simulink model "elaborated_design"  (Simulink 7.0)
settings: Solver=ode45  SolverMode=SingleTasking  StartTime=0.0  StopTime=24/3000  RelTol=1e-6
PreLoadFcn:
  | load one_stage.mat
  | load multi_stage.mat
  | generate_fir_lut
undefined symbols (not defined in the file or in its folder): hm, lut_matrix
libraries: simulink x9, dspmlti4 x4, simulink_extras x2, dspsigops x1
(part 2 of 2)

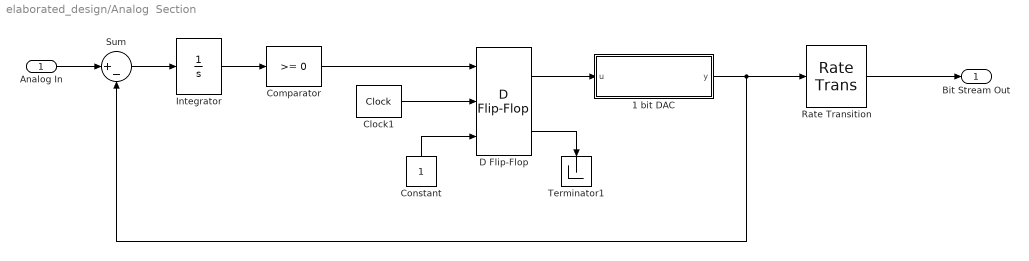
== system elaborated_design/Analog  Section ==
  Analog In : Inport  OutDataType=sfix(16)  OutScaling=2^0
  1 bit DAC : Stateflow chart
  Clock1 : simulink_extras/Flip Flops/Clock  SystemSampleTime=-1  MaskParam1=1/(48e3*64)
  Comparator : simulink/Logic and Bit Operations/Compare To Zero  SystemSampleTime=-1  relop=>=  LogicOutDataTypeMode=boolean  ZeroCross=off
  Constant : Constant  Orientation=up  OutDataType=sfix(16)  OutScaling=2^0  SampleTime=0
  D Flip-Flop : simulink_extras/Flip Flops/D Flip-Flop  SystemSampleTime=-1
  Integrator : Integrator
  Rate Transition : RateTransition  OutPortSampleTime=1/(48e3*64)
  Sum : Sum  Inputs=|+-  OutDataType=sfix(16)  OutScaling=2^0
  Terminator1 : Terminator
      settings: Orientation=down
  Bit Stream Out : Outport  DataType=double  OutDataType=sfix(16)  OutScaling=2^0
  wires:
  Sum/1 -> Integrator/1
  Integrator/1 -> Comparator/1
  Comparator/1 -> D Flip-Flop/1
  Analog In/1 -> Sum/1
  D Flip-Flop/2 -> Terminator1/1
  Clock1/1 -> D Flip-Flop/2
  D Flip-Flop/1 -> 1 bit DAC/1(u)
  Constant/1 -> D Flip-Flop/3
  1 bit DAC/1(y) -> Sum/2, Rate Transition/1
  Rate Transition/1 -> Bit Stream Out/1

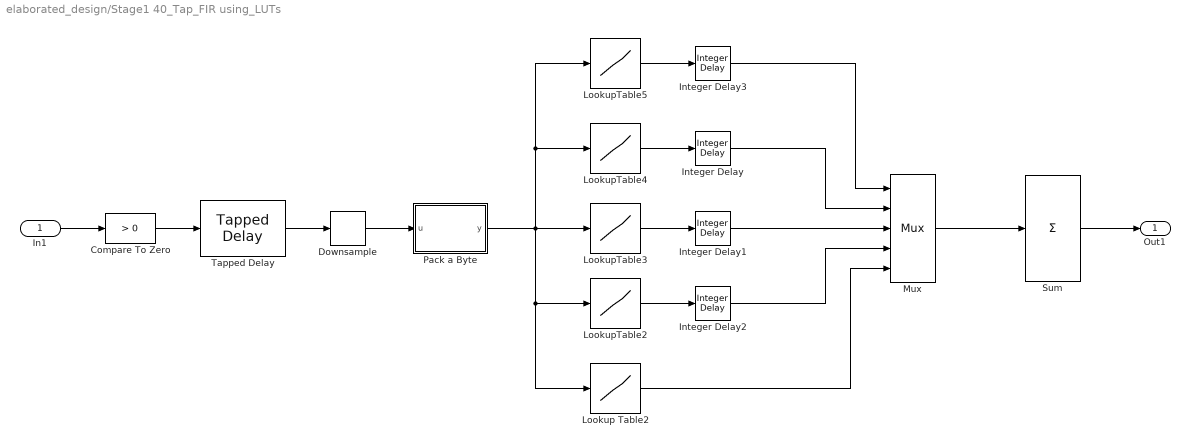
== system elaborated_design/Stage1 40_Tap_FIR using_LUTs ==
  In1 : Inport  OutDataType=sfix(16)  OutScaling=2^0
  Compare To Zero : simulink/Logic and Bit Operations/Compare To Zero  SystemSampleTime=-1  relop=>  LogicOutDataTypeMode=boolean  ZeroCross=off
  Downsample : dspsigops/Downsample  N=8  phase=0  ic=0  smode=Allow multirate  fmode=Maintain input frame size
  Integer Delay : simulink/Discrete/Integer Delay  vinit=0.0  samptime=-1  NumDelays=3
  Integer Delay1 : simulink/Discrete/Integer Delay  vinit=0.0  samptime=-1  NumDelays=2
  Integer Delay2 : simulink/Discrete/Integer Delay  vinit=0.0  samptime=-1  NumDelays=1
  Integer Delay3 : simulink/Discrete/Integer Delay  vinit=0.0  samptime=-1  NumDelays=4
  Lookup Table2 : Lookup  InputValues=[0:255]  Table=[lut_matrix(1,:)]  OutDataTypeMode=double  OutDataType=sfix(16)  OutScaling=2^0
  LookupTable2 : Lookup  InputValues=[0:255]  Table=lut_matrix(2,:)  OutDataTypeMode=double  OutDataType=sfix(16)  OutScaling=2^0
  LookupTable3 : Lookup  InputValues=[0:255]  Table=lut_matrix(3,:)  OutDataTypeMode=double  OutDataType=sfix(16)  OutScaling=2^0
  LookupTable4 : Lookup  InputValues=[0:255]  Table=lut_matrix(4,:)  OutDataTypeMode=double  OutDataType=sfix(16)  OutScaling=2^0
  LookupTable5 : Lookup  InputValues=[0:255]  Table=lut_matrix(5,:)  OutDataTypeMode=double  OutDataType=sfix(16)  OutScaling=2^0
  Mux : Mux  Inputs=5
  Pack a Byte : Stateflow chart
  Sum : Sum  Inputs=+  OutDataTypeMode=double  OutDataType=fixdt(1,13,10)  SaturateOnIntegerOverflow=on
  Tapped Delay : simulink/Discrete/Tapped Delay  vinit=0  samptime=-1  NumDelays=8  DelayOrder=Oldest  includeCurrent=off
  Out1 : Outport  OutDataType=sfix(16)  OutScaling=2^0
  wires:
  LookupTable4/1 -> Integer Delay/1
  LookupTable3/1 -> Integer Delay1/1
  LookupTable2/1 -> Integer Delay2/1
  LookupTable5/1 -> Integer Delay3/1
  In1/1 -> Compare To Zero/1
  Tapped Delay/1 -> Downsample/1
  Downsample/1 -> Pack a Byte/1(u)
  Pack a Byte/1(y) -> LookupTable5/1, LookupTable4/1, LookupTable3/1, LookupTable2/1, Lookup Table2/1
  Compare To Zero/1 -> Tapped Delay/1
  Mux/1 -> Sum/1
  Sum/1 -> Out1/1
  Integer Delay3/1 -> Mux/1
  Integer Delay/1 -> Mux/2
  Integer Delay1/1 -> Mux/3
  Integer Delay2/1 -> Mux/4
  Lookup Table2/1 -> Mux/5

== matlab function Analog Section/1 bit DAC ==
  data: u input inherited; y output inherited
function y = DAC_1_bit(u)
% This block supports an embeddable subset of the MATLAB language.
% See the help menu for details.

% This code converts boolean input to a bipolar output (double precision).
% We chose to write this in EML function block but we could have also done 
% this with simulink blocks.

y=-1+2*u;

== matlab function Stage1 40_Tap_FIR using_LUTs/Pack a Byte ==
  data: u input inherited; y output uint8
function y = fcn(u)
% This block supports an embeddable subset of the MATLAB language.
% See the help menu for details.

% This function packs eight bits into one byte.
y = uint8(0);
for k = 1:8
    y = bitset(y,k,u(k));
end
